simulink model "CLIK"  (R2022b)
settings: Solver=VariableStepAuto  StartTime=0.0  StopTime=40  RelTol=1e-3
values from neighbouring files (symbols this model uses):
  T = T_A * T_B    [DH_dinamica.m]    (also in traiettoria_script.m = 0.001)
  theta1_0 = pi/2 - angolo    [CLIK_script.m]
  theta2_0 = 2*angolo    [CLIK_script.m]
undefined symbols (not defined in the file or in its folder): DiscIntNeverNeededParam
libraries: simulink x3
settings Model: Creator=Michele  LastModifiedBy=Michele
settings DataIOCC: ReturnWorkspaceOutputs=off

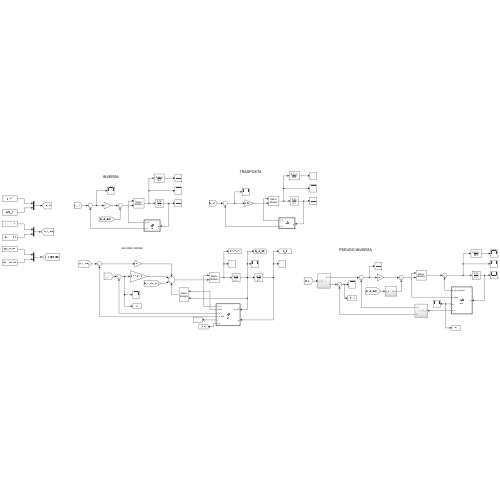
[thumbnail: Simulink's stored preview of the top-level diagram]
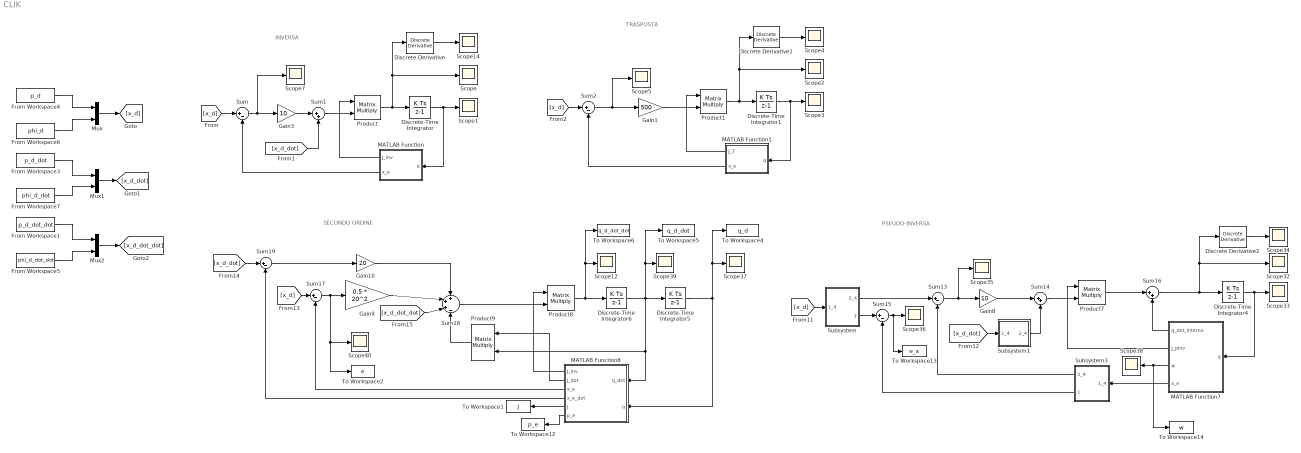
== system CLIK ==
  note: INVERSA
  note: TRASPOSTA
  note: SECONDO ORDINE
  note: PSEUDO-INVERSA
  Discrete Derivative : simulink/Discrete/Discrete Derivative  gainval=1.0  ICPrevScaledInput=[0 0 0 0]'  OutMin=[]  OutMax=[]  OutDataType=fixdt(1, 16)  OutScaling=2^-10  DoSatur=off
  Discrete Derivative1 : simulink/Discrete/Discrete Derivative  gainval=1.0  ICPrevScaledInput=[0 0 0 0]'  OutMin=[]  OutMax=[]  OutDataType=fixdt(1, 16)  OutScaling=2^-10  DoSatur=off
  Discrete Derivative2 : simulink/Discrete/Discrete Derivative  gainval=1.0  ICPrevScaledInput=[0 0 0 0]'  OutMin=[]  OutMax=[]  OutDataType=fixdt(1, 16)  OutScaling=2^-10  DoSatur=off
  Discrete-Time Integrator{,1,4..5} (4 alike) : DiscreteIntegrator  InitialCondition=[theta1_0 theta2_0 -0.25 0]'  SampleTime=-1  ICPrevOutput=DiscIntNeverNeededParam  ICPrevScaledInput=DiscIntNeverNeededParam
  Discrete-Time Integrator6 : DiscreteIntegrator  InitialCondition=[0 0 0 0]'  SampleTime=-1  ICPrevOutput=DiscIntNeverNeededParam  ICPrevScaledInput=DiscIntNeverNeededParam
  From Workspace1 : FromWorkspace  VariableName=p_d_dot_dot  SampleTime=T
  From Workspace3 : FromWorkspace  VariableName=p_d_dot  SampleTime=T
  From Workspace4 : FromWorkspace  VariableName=p_d  SampleTime=T
  From Workspace5 : FromWorkspace  VariableName=phi_d_dot_dot  SampleTime=T
  From Workspace6 : FromWorkspace  VariableName=phi_d  SampleTime=T
  From Workspace7 : FromWorkspace  VariableName=phi_d_dot  SampleTime=T
  Gain1 : Gain  Gain=500
  Gain10 : Gain  Gain=20
  Gain3 : Gain  Gain=10
  Gain8 : Gain  Gain=10
  Gain9 : Gain  Gain=0.5 * 20^2
  MATLAB Function : MATLAB Function  TreatAsAtomicUnit=on
  MATLAB Function1 : MATLAB Function  TreatAsAtomicUnit=on
  MATLAB Function7 : MATLAB Function  TreatAsAtomicUnit=on
  MATLAB Function8 : MATLAB Function  TreatAsAtomicUnit=on
  Mux : Mux  Inputs=2
  Mux1 : Mux  Inputs=2
  Mux2 : Mux  Inputs=2
  Product{,1,7..9} (5 alike) : Product  Multiplication=Matrix(*)
  Scope{,1..5,7,12,14,32..40} (18 alike) : Scope
  Subsystem : Subsystem
  Subsystem1 : Subsystem
  Subsystem3 : Subsystem
  Sum{,2,13,15,17,19} (6 alike) : Sum  Inputs=|+-
  Sum1 : Sum  Inputs=|++
  Sum14 : Sum  Inputs=|++
  Sum16 : Sum  Inputs=|++
  Sum18 : Sum  Inputs=+++-
  To Workspace1 : ToWorkspace  VariableName=J  SaveFormat=Structure With Time  SampleTime=-1
  To Workspace12 : ToWorkspace  VariableName=p_e  SaveFormat=Structure With Time  SampleTime=-1
  To Workspace13 : ToWorkspace  VariableName=e_x  SaveFormat=Structure With Time  SampleTime=-1
  To Workspace14 : ToWorkspace  VariableName=w  SaveFormat=Structure With Time  SampleTime=-1
  To Workspace2 : ToWorkspace  VariableName=e  SaveFormat=Structure With Time  SampleTime=-1
  To Workspace4 : ToWorkspace  VariableName=q_d  SaveFormat=Structure With Time  SampleTime=-1
  To Workspace5 : ToWorkspace  VariableName=q_d_dot  SaveFormat=Structure With Time  SampleTime=-1
  To Workspace6 : ToWorkspace  VariableName=q_d_dot_dot  SaveFormat=Structure With Time  SampleTime=-1
  wires:
  MATLAB Function/2(x_e) -> Sum/2
  Sum/1 -> Gain3/1, Scope7/1
  [x_d_dot] -> Sum1/2
  Gain3/1 -> Sum1/1
  Sum1/1 -> Product/2
  MATLAB Function/1(J_inv) -> Product/1
  Discrete Derivative/1 -> Scope14/1
  [x_d] -> Sum/1
  Product/1 -> Discrete-Time Integrator/1, Discrete Derivative/1, Scope/1
  Gain8/1 -> Sum14/1
  Sum16/1 -> Discrete Derivative2/1, Scope32/1, Discrete-Time Integrator4/1
  Discrete Derivative2/1 -> Scope34/1
  MATLAB Function7/3(w) -> To Workspace14/1, Scope38/1
  Product7/1 -> Sum16/1
  MATLAB Function7/2(J_pinv) -> Product7/1
  Sum13/1 -> Gain8/1, Scope35/1
  Discrete-Time Integrator4/1 -> MATLAB Function7/1(q), Scope33/1
  MATLAB Function7/1(q_dot_interno) -> Sum16/2
  [x_d] -> Subsystem/1(1_4)
  Subsystem/1(2_4) -> Sum13/1
  MATLAB Function7/4(x_e) -> Subsystem3/1(1_4)
  [x_d_dot] -> Subsystem1/1(1_4)
  Sum14/1 -> Product7/2
  Subsystem1/1(2_4) -> Sum14/2
  Subsystem/2(1) -> Sum15/1
  Sum15/1 -> To Workspace13/1, Scope36/1
  Discrete-Time Integrator6/1 -> To Workspace5/1, Scope39/1, Discrete-Time Integrator5/1, Product9/2, MATLAB Function8/1(q_dot)
  MATLAB Function8/3(x_e) -> Sum17/2
  Sum18/1 -> Product8/2
  MATLAB Function8/2(J_dot) -> Product9/1
  Product8/1 -> Discrete-Time Integrator6/1, To Workspace6/1, Scope12/1
  Discrete-Time Integrator5/1 -> To Workspace4/1, Scope37/1, MATLAB Function8/2(q)
  Gain9/1 -> Sum18/2
  [x_d] -> Sum17/1
  Gain10/1 -> Sum18/1
  MATLAB Function8/4(x_e_dot) -> Sum19/2
  [x_d_dot] -> Sum19/1
  Sum17/1 -> To Workspace2/1, Scope40/1, Gain9/1
  Sum19/1 -> Gain10/1
  [x_d_dot_dot] -> Sum18/3
  Product9/1 -> Sum18/4
  MATLAB Function8/1(J_inv) -> Product8/1
  Product1/1 -> Discrete-Time Integrator1/1, Discrete Derivative1/1, Scope2/1
  Discrete-Time Integrator1/1 -> MATLAB Function1/1(q), Scope3/1
  Gain1/1 -> Product1/2
  MATLAB Function1/2(x_e) -> Sum2/2
  MATLAB Function1/1(J_T) -> Product1/1
  Discrete Derivative1/1 -> Scope4/1
  [x_d] -> Sum2/1
  Sum2/1 -> Gain1/1, Scope5/1
  Subsystem3/1(2_4) -> Sum13/2
  Subsystem3/2(1) -> Sum15/2
  MATLAB Function8/5(J) -> To Workspace1/1
  MATLAB Function8/6(p_e) -> To Workspace12/1
  Discrete-Time Integrator/1 -> Scope1/1, MATLAB Function/1(q)
  Mux1/1 -> [x_d_dot]
  From Workspace3/1 -> Mux1/1
  Mux/1 -> [x_d]
  From Workspace7/1 -> Mux1/2
  From Workspace5/1 -> Mux2/2
  From Workspace1/1 -> Mux2/1
  Mux2/1 -> [x_d_dot_dot]
  From Workspace4/1 -> Mux/1
  From Workspace6/1 -> Mux/2

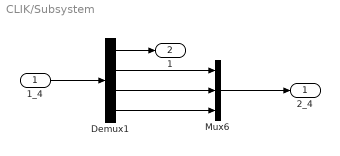
== system CLIK/Subsystem ==
  1_4 : Inport
  Demux1 : Demux
  Mux6 : Mux  Inputs=3
  2_4 : Outport
  1 : Outport  Port=2
  wires:
  Mux6/1 -> 2_4/1
  Demux1/4 -> Mux6/3
  1_4/1 -> Demux1/1
  Demux1/2 -> Mux6/1
  Demux1/3 -> Mux6/2
  Demux1/1 -> 1/1

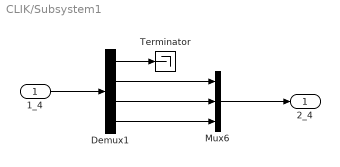
== system CLIK/Subsystem1 ==
  1_4 : Inport
  Demux1 : Demux
  Mux6 : Mux  Inputs=3
  Terminator : Terminator
  2_4 : Outport
  wires:
  Mux6/1 -> 2_4/1
  Demux1/4 -> Mux6/3
  1_4/1 -> Demux1/1
  Demux1/2 -> Mux6/1
  Demux1/3 -> Mux6/2
  Demux1/1 -> Terminator/1

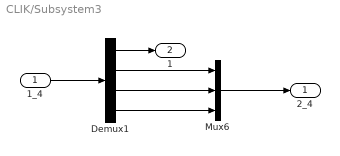
== system CLIK/Subsystem3 ==
  1_4 : Inport
  Demux1 : Demux
  Mux6 : Mux  Inputs=3
  2_4 : Outport
  1 : Outport  Port=2
  wires:
  Mux6/1 -> 2_4/1
  Demux1/4 -> Mux6/3
  1_4/1 -> Demux1/1
  Demux1/2 -> Mux6/1
  Demux1/3 -> Mux6/2
  Demux1/1 -> 1/1

== matlab function CLIK/MATLAB Function1 ==
  data: J_T output; q input; x_e output
function [J_T,x_e] = kin(q)

    q1 = q(1); q2 = q(2); q3 = q(3); q4 = q(4);

    J = [- sin(q1)/2 - (cos(q1)*sin(q2))/2 - (cos(q2)*sin(q1))/2, - (cos(q1)*sin(q2))/2 - (cos(q2)*sin(q1))/2, 0, 0;
           cos(q1)/2 + (cos(q1)*cos(q2))/2 - (sin(q1)*sin(q2))/2,   (cos(q1)*cos(q2))/2 - (sin(q1)*sin(q2))/2, 0, 0;
                                                               0,                                           0, 1, 0;
                                                               0,                                           0, 0, 1];

    x_e = [cos(q1)/2 + (cos(q1)*cos(q2))/2 - (sin(q1)*sin(q2))/2;
           sin(q1)/2 + (cos(q1)*sin(q2))/2 + (cos(q2)*sin(q1))/2;
                                                   q3;
                                                   q4];

    J_T = transpose(J);
end

== matlab function CLIK/MATLAB Function ==
  data: J_inv output; q input; x_e output
function [J_inv,x_e] = kin(q)
    
    q1 = q(1); q2 = q(2); q3 = q(3); q4 = q(4);

    J = [- sin(q1)/2 - (cos(q1)*sin(q2))/2 - (cos(q2)*sin(q1))/2, - (cos(q1)*sin(q2))/2 - (cos(q2)*sin(q1))/2, 0, 0;
           cos(q1)/2 + (cos(q1)*cos(q2))/2 - (sin(q1)*sin(q2))/2,   (cos(q1)*cos(q2))/2 - (sin(q1)*sin(q2))/2, 0, 0;
                                                               0,                                           0, 1, 0;
                                                               0,                                           0, 0, 1];

    x_e = [cos(q1)/2 + (cos(q1)*cos(q2))/2 - (sin(q1)*sin(q2))/2;
           sin(q1)/2 + (cos(q1)*sin(q2))/2 + (cos(q2)*sin(q1))/2;
                                                   q3;
                                                   q4];
    
    J_inv= inv(J);
end

== matlab function CLIK/MATLAB Function7 ==
  data: q_dot_interno output; J_pinv output; w output; q input; x_e output
function [q_dot_interno,J_pinv,w,x_e] = kin(q)

    q1 = q(1); q2 = q(2); q3 = q(3); q4 = q(4);

    J = [- sin(q1)/2 - (cos(q1)*sin(q2))/2 - (cos(q2)*sin(q1))/2, - (cos(q1)*sin(q2))/2 - (cos(q2)*sin(q1))/2, 0, 0;
           cos(q1)/2 + (cos(q1)*cos(q2))/2 - (sin(q1)*sin(q2))/2,   (cos(q1)*cos(q2))/2 - (sin(q1)*sin(q2))/2, 0, 0;
                                                               0,                                           0, 1, 0;
                                                               0,                                           0, 0, 1];

    x_e = [cos(q1)/2 + (cos(q1)*cos(q2))/2 - (sin(q1)*sin(q2))/2;
           sin(q1)/2 + (cos(q1)*sin(q2))/2 + (cos(q2)*sin(q1))/2;
                                                   q3;
                                                   q4];
    J = J(2:end,:);

    J_pinv = pinv(J);

    P = eye(4) - J_pinv*J;
    q_dot_interno = P * 5 * [0 cos(q(2)) 0 0]';

    w = sqrt(det(J*J'));
end

== matlab function CLIK/MATLAB Function8 ==
  data: J_inv output; J_dot output; x_e output; x_e_dot output; q_dot input; q input; J output; p_e output
function [J_inv,J_dot,x_e,x_e_dot,J,p_e] = kin(q_dot,q)

    q1 = q(1); q2 = q(2); q3 = q(3); q4 = q(4);
    q_dot1 = q_dot(1); q_dot2 = q_dot(2); q_dot3 = q_dot(3); q_dot4 = q_dot(4);

    J = [- sin(q1)/2 - (cos(q1)*sin(q2))/2 - (cos(q2)*sin(q1))/2, - (cos(q1)*sin(q2))/2 - (cos(q2)*sin(q1))/2, 0, 0;
           cos(q1)/2 + (cos(q1)*cos(q2))/2 - (sin(q1)*sin(q2))/2,   (cos(q1)*cos(q2))/2 - (sin(q1)*sin(q2))/2, 0, 0;
                                                               0,                                           0, 1, 0;
                                                               0,                                           0, 0, 1];

    x_e = [cos(q1)/2 + (cos(q1)*cos(q2))/2 - (sin(q1)*sin(q2))/2;
           sin(q1)/2 + (cos(q1)*sin(q2))/2 + (cos(q2)*sin(q1))/2;
                                                   q3;
                                                   q4];
    
    J_inv = inv(J);

    J_dot = [- q_dot2*((cos(q1)*cos(q2))/2 - (sin(q1)*sin(q2))/2) - q_dot1*(cos(q1)/2 + (cos(q1)*cos(q2))/2 - (sin(q1)*sin(q2))/2), (q_dot1*cos(q1))/2 - q_dot1*(cos(q1)/2 + (cos(q1)*cos(q2))/2 - (sin(q1)*sin(q2))/2) - q_dot2*((cos(q1)*cos(q2))/2 - (sin(q1)*sin(q2))/2), 0, 0;
             - q_dot2*((cos(q1)*sin(q2))/2 + (cos(q2)*sin(q1))/2) - q_dot1*(sin(q1)/2 + (cos(q1)*sin(q2))/2 + (cos(q2)*sin(q1))/2), (q_dot1*sin(q1))/2 - q_dot1*(sin(q1)/2 + (cos(q1)*sin(q2))/2 + (cos(q2)*sin(q1))/2) - q_dot2*((cos(q1)*sin(q2))/2 + (cos(q2)*sin(q1))/2), 0, 0;
                                                                                                                                 0,                                                                                                                                        0, 0, 0;
                                                                                                                                 0,                                                                                                                                        0, 0, 0];

    x_e_dot = J*q_dot;

    p_e = x_e(1:3);
end
